simulink model "PubIfDecisionTOS_MDL"  (R2020b)
settings: configuration reference "DspaceConfig" (kept outside this file)
PostLoadFcn:
  | if any(exist('dsrtsu_mdlpostloadfcn', 'file') ~= 0), dsrtsu_mdlpostloadfcn('Execute', bdroot); end
InitFcn:
  | , if any(exist('dsmpb_private', 'file') ~= 0), dsmpb_private('dsmpb_mdlclblib', 'Init', bdroot); end,
undefined symbols (not defined in the file or in its folder): C_TOS_ACCEgoRAxletoFbumplength_m, C_TOS_ACCTargetFront_Flag, C_TOS_AEBJAPedObjDxThre_Val, C_TOS_AEBJAPedObjDyThre_Val, C_TOS_AEBJATargetSize_Val, C_TOS_AEBJAVehObjDxThre_Val, C_TOS_AEBJAVehObjDyThre_Val, C_TOS_AEBJuncPedTargetSize_Val, C_TOS_AEBLatObjDxThre_Val, C_TOS_AEBLatPedDyThre_Val, C_TOS_AEBLatTargetSize_Val, C_TOS_AEBLongTargetInEgoFront_Flag, C_TOS_axAbsGround_Parameter, C_TOS_CameraConfirmedFlag, C_TOS_CNsubjWidth, C_TOS_CurrentLaneCoreMinWidth_Val, C_TOS_CutInProb_Val_Zero, C_TOS_CutOutProb_Val_Zero, C_TOS_D2R_Val, C_TOS_DefaultValueObjectToCenterLine_dy, C_TOS_EgoCarWidth_Val, C_TOS_EgoDxRefPoint_m, C_TOS_EgoRAxletoFbumplength_m, C_TOS_HalfWidthVehicle_Con, C_TOS_HWA_CurrentLaneFlag, C_TOS_HWA_LeftLaneFlag, C_TOS_HWA_MovingDir_Vaild, C_TOS_HWA_MovState_Vaild, C_TOS_HWA_RightLaneFlag, C_TOS_LaneLineCourseErrorFront, C_TOS_LaneLineCourseErrorRear, C_TOS_MotorbikeDefaultWidth_m, C_TOS_NumberOfEffectiveTargets, C_TOS_Obj_Age_Val, C_TOS_Objdx_Constraint_Val, C_TOS_ObjectDefaultWidth_m, C_TOS_ObjInCurrentLane_Val, C_TOS_ObjInCurrentLaneValid, C_TOS_ObjInLeftLaneValid, C_TOS_ObjInRightLaneValid, C_TOS_ObjNotInCurrentLane_Val, C_TOS_ObjNotREElementType, C_TOS_ObjPredictDis_dy_ConstantVal_Zeros, C_TOS_ObjToCenterLine_ConstantVal_Zeros, C_TOS_OFMObjIDInvilad_Val, C_TOS_PIL_LatDisCons_Val_zero, C_TOS_PIL_ObjectCutInFlag_b, C_TOS_PIL_ObjectCutOutFlag_b, C_TOS_PIL_ObjLaneProb_al_Val, C_TOS_PP_ObjFusType_FC_Confirm_b, C_TOS_PP_ObjFusType_FC_FR_Confirm_b, C_TOS_PP_ObjFusType_FR_Confirm_b, C_TOS_RE_80BoolDefault_Val, C_TOS_RE_80Single181Default_Val, C_TOS_RE_80Single255Default_Val, C_TOS_RE_80Uint8Default_Val, C_TOS_RE_D2R, C_TOS_RE_D_180_Val, C_TOS_RE_InvalidObjectID_Val, C_TOS_RE_InvalidTargetChainDir_Val ... (+142)
libraries: simulink x1650, TOS_LIB x361, canfdmsglib x14
(part 60 of 69)

== system PubIfDecisionTOS_MDL/TOS_20201112/TOS_2012080320/TOS/AEB/TOS_AEBLong/AEBLong_Confirm/AEBLong/AEBLong_TrgConfirm/AEBLongTrgJudg/TOS_AEBLong_TargetMovingDir/ObjMovingDirSignalProcessing1/Oncoming_MovingDir_StrightLane/OncomingVYCondition ==
  Object_MappingVY : Inport
  Object_MappingVX : Inport  Port=2
  Abs : Abs
  Abs1 : Abs
  Relational Operator : RelationalOperator  Operator=<  OutDataTypeStr=boolean  RndMeth=Nearest
  VYThre_BaseVX : Lookup_n-D  NumberOfTableDimensions=1  BreakpointsForDimension1=[0,8.3,16.67,25,33.3,40]  Table=[0,3.5,5,7.5,9.3,9.3]  InternalRulePriority=Speed  RndMeth=Simplest  InputSameDT=on
  OncomingVYflg : Outport
  wires:
  Object_MappingVX/1 -> Abs1/1
  Relational Operator/1 -> OncomingVYflg/1
  Abs/1 -> Relational Operator/1
  VYThre_BaseVX/1 -> Relational Operator/2
  Object_MappingVY/1 -> Abs/1
  Abs1/1 -> VYThre_BaseVX/1

== system PubIfDecisionTOS_MDL/TOS_20201112/TOS_2012080320/TOS/AEB/TOS_AEBLong/AEBLong_Confirm/AEBLong/AEBLong_TrgConfirm/AEBLongTrgJudg/TOS_AEBLong_TargetMovingDir/ObjMovingDirSignalProcessing1/Oncoming_MovingDir_StrightLane/OncomingVYVXAngle ==
  Object_VXVYAngle : Inport
  135 : Constant  Value=P_TOS_ObjLatCroYawAngMaxThre_Val  OutDataTypeStr=single
      settings: AttributesFormatString=P_TOS_ObjLatCroYawAngMaxThre_Val = 135
  45 : Constant  Value=P_TOS_ObjOncomingYawAngMaxThre_Val  OutDataTypeStr=single
      settings: AttributesFormatString=P_TOS_ObjOncomingYawAngMaxThre_Val = 180
  Abs : Abs
  Logical Operator : Logic  AllPortsSameDT=off  OutDataTypeStr=boolean
  Relational Operator : RelationalOperator  Operator=>  OutDataTypeStr=boolean  RndMeth=Nearest
  Relational Operator1 : RelationalOperator  Operator=<=  OutDataTypeStr=boolean  RndMeth=Nearest
  OncomingVYVXAngleFlg : Outport
  wires:
  Logical Operator/1 -> OncomingVYVXAngleFlg/1
  Relational Operator1/1 -> Logical Operator/2
  45/1 -> Relational Operator1/2
  135/1 -> Relational Operator/2
  Abs/1 -> Relational Operator1/1, Relational Operator/1
  Relational Operator/1 -> Logical Operator/1
  Object_VXVYAngle/1 -> Abs/1

== system PubIfDecisionTOS_MDL/TOS_20201112/TOS_2012080320/TOS/AEB/TOS_AEBLong/AEBLong_Confirm/AEBLong/AEBLong_TrgConfirm/AEBLongTrgJudg/TOS_AEBLong_TargetMovingDir/ObjMovingDirSignalProcessing1/Oncoming_MovingDir_StrightLane1/CrossingVXCondition ==
  Object_MappingVX : Inport
  Object_MappingVY : Inport  Port=2
  Abs : Abs
  Abs1 : Abs
  Relational Operator : RelationalOperator  Operator=<  OutDataTypeStr=boolean  RndMeth=Nearest
  VXThre_BaseVY : Lookup_n-D  NumberOfTableDimensions=1  BreakpointsForDimension1=[0,8.3,16.67,25,33.3,40]  Table=[0,2.1,4.5,6.7,9,9]  InternalRulePriority=Speed  RndMeth=Simplest  InputSameDT=on
  CrossingVXflg : Outport
  wires:
  Object_MappingVX/1 -> Abs/1
  VXThre_BaseVY/1 -> Relational Operator/2
  Abs/1 -> Relational Operator/1
  Relational Operator/1 -> CrossingVXflg/1
  Object_MappingVY/1 -> Abs1/1
  Abs1/1 -> VXThre_BaseVY/1

== system PubIfDecisionTOS_MDL/TOS_20201112/TOS_2012080320/TOS/AEB/TOS_AEBLong/AEBLong_Confirm/AEBLong/AEBLong_TrgConfirm/AEBLongTrgJudg/TOS_AEBLong_TargetMovingDir/ObjMovingDirSignalProcessing1/Oncoming_MovingDir_StrightLane1/CrossingVYCondition ==
  note: VYThre
  Object_MappingVY : Inport
  Object_DX : Inport  Port=2
  Object_DY : Inport  Port=3
  Abs : Abs
  Abs1 : Abs
  Abs2 : Abs
  Product : Product
  Relational Operator1 : RelationalOperator  Operator=>  OutDataTypeStr=boolean  RndMeth=Nearest
  VYThre_BaseDX : Lookup_n-D  NumberOfTableDimensions=1  BreakpointsForDimension1=[0,30,60,90,120,150]  Table=[0,0.5,0.7,0.8,0.9,0.9]  InternalRulePriority=Speed  RndMeth=Simplest  InputSameDT=on
  VYThre_BaseDY : Lookup_n-D  NumberOfTableDimensions=1  BreakpointsForDimension1=[0,5,10,15,20,30,50]  Table=[1,1.1,1.12,1.15,1.2,1.2,1.2]  InternalRulePriority=Speed  RndMeth=Simplest  InputSameDT=on
  CrossingVYFlg : Outport
  wires:
  Object_MappingVY/1 -> Abs/1
  Product/1 -> Relational Operator1/2
  VYThre_BaseDX/1 -> Product/1
  Relational Operator1/1 -> CrossingVYFlg/1
  Object_DX/1 -> Abs1/1
  VYThre_BaseDY/1 -> Product/2
  Object_DY/1 -> Abs2/1
  Abs/1 -> Relational Operator1/1
  Abs1/1 -> VYThre_BaseDX/1
  Abs2/1 -> VYThre_BaseDY/1

== system PubIfDecisionTOS_MDL/TOS_20201112/TOS_2012080320/TOS/AEB/TOS_AEBLong/AEBLong_Confirm/AEBLong/AEBLong_TrgConfirm/AEBLongTrgJudg/TOS_AEBLong_TargetMovingDir/ObjMovingDirSignalProcessing1/Oncoming_MovingDir_StrightLane1/CrossingVYVXAngle ==
  Object_VYVXAngle : Inport
  135.0 : Constant  Value=P_TOS_ObjLatCroYawAngMaxThre_Val  OutDataTypeStr=single
      settings: AttributesFormatString=P_TOS_ObjLatCroYawAngMaxThre_Val = 135
  45.00 : Constant  Value=P_TOS_ObjLatCroYawAngMinThre_Val  OutDataTypeStr=single
      settings: AttributesFormatString=P_TOS_ObjLatCroYawAngMinThre_Val = 45
  Abs : Abs
  Logical Operator : Logic  AllPortsSameDT=off  OutDataTypeStr=boolean
  Relational Operator : RelationalOperator  Operator=>  OutDataTypeStr=boolean  RndMeth=Nearest
  Relational Operator1 : RelationalOperator  Operator=<=  OutDataTypeStr=boolean  RndMeth=Nearest
  CrossingVYVXAngleFlg : Outport
  wires:
  Object_VYVXAngle/1 -> Abs/1
  Relational Operator/1 -> Logical Operator/1
  Abs/1 -> Relational Operator/1, Relational Operator1/1
  45.00/1 -> Relational Operator/2
  135.0/1 -> Relational Operator1/2
  Relational Operator1/1 -> Logical Operator/2
  Logical Operator/1 -> CrossingVYVXAngleFlg/1

== system PubIfDecisionTOS_MDL/TOS_20201112/TOS_2012080320/TOS/LC_LCKie_ELK/TOS_HWA/CurrentLane/HWA_CurrentLane_Target/HWA_CLF_Target_1/HWA_CLF_Target/HWA_CLF_Target/HWA_CLF_FusionTypeConfirm/TOS_ACCFusionTypeAborDly/If Action Subsystem ==
  HWA_CLF_FusionType : Inport
  Action Port : ActionPort  ActionPortLabel=else
  HWA_CLF_FusionTypeFilt : Outport
  wires:
  HWA_CLF_FusionType/1 -> HWA_CLF_FusionTypeFilt/1

== system PubIfDecisionTOS_MDL/TOS_20201112/TOS_2012080320/TOS/LC_LCKie_ELK/TOS_HWA/CurrentLane/HWA_CurrentLane_Target/HWA_CLF_Target_1/HWA_CLF_Target/HWA_CLF_Target/HWA_CLF_FusionTypeConfirm/TOS_ACCFusionTypeAborDly/If Action Subsystem1 ==
  HWA_CLF_FusionType : Inport
  Action Port : ActionPort  ActionPortLabel=if(u1)
  Constant : Constant  Value=0.15
  Constant4 : Constant  Value=0.05
  StateDelayAbortion : TOS_LIB/StateDelayAbortion  SystemSampleTime=-1  VariantActivationTime=update diagram  Latency=0  AutoFrameSizeCalculation=off
  HWA_CLF_FusionTypeFilt : Outport
  wires:
  StateDelayAbortion/1 -> HWA_CLF_FusionTypeFilt/1
  Constant/1 -> StateDelayAbortion/2
  Constant4/1 -> StateDelayAbortion/3
  HWA_CLF_FusionType/1 -> StateDelayAbortion/1

== system PubIfDecisionTOS_MDL/TOS_20201112/TOS_2012080320/TOS/LC_LCKie_ELK/TOS_HWA/CurrentLane/HWA_CurrentLane_Target/HWA_CLF_Target_1/HWA_CLF_Target/HWA_CLF_Target/HWA_CLF_ObjTypeConfirm/TOS_ObjTypeAborDly/If Action Subsystem ==
  FusionType : Inport
  Action Port : ActionPort  ActionPortLabel=else
  FusionTypeFilt : Outport
  wires:
  FusionType/1 -> FusionTypeFilt/1

== system PubIfDecisionTOS_MDL/TOS_20201112/TOS_2012080320/TOS/LC_LCKie_ELK/TOS_HWA/CurrentLane/HWA_CurrentLane_Target/HWA_CLF_Target_1/HWA_CLF_Target/HWA_CLF_Target/HWA_CLF_ObjTypeConfirm/TOS_ObjTypeAborDly/If Action Subsystem1 ==
  FusionType : Inport
  Action Port : ActionPort  ActionPortLabel=if(u1)
  Constant : Constant  Value=0.15
  Constant4 : Constant  Value=0.05
  StateDelayAbortion : TOS_LIB/StateDelayAbortion  SystemSampleTime=-1  VariantActivationTime=update diagram  Latency=0  AutoFrameSizeCalculation=off
  FusionTypeFilt : Outport
  wires:
  StateDelayAbortion/1 -> FusionTypeFilt/1
  Constant/1 -> StateDelayAbortion/2
  Constant4/1 -> StateDelayAbortion/3
  FusionType/1 -> StateDelayAbortion/1

== system PubIfDecisionTOS_MDL/TOS_20201112/TOS_2012080320/TOS/LC_LCKie_ELK/TOS_HWA/CurrentLane/HWA_CurrentLane_Target/HWA_CLF_Target_1/HWA_CLF_Target/HWA_CLF_Target/HWA_CLF_ObstacleProbConfirm/ObstacleProbAborDly/If Action Subsystem ==
  FusionType : Inport
  Action Port : ActionPort  ActionPortLabel=else
  FusionTypeFilt : Outport
  wires:
  FusionType/1 -> FusionTypeFilt/1

== system PubIfDecisionTOS_MDL/TOS_20201112/TOS_2012080320/TOS/LC_LCKie_ELK/TOS_HWA/CurrentLane/HWA_CurrentLane_Target/HWA_CLF_Target_1/HWA_CLF_Target/HWA_CLF_Target/HWA_CLF_ObstacleProbConfirm/ObstacleProbAborDly/If Action Subsystem1 ==
  FusionType : Inport
  Action Port : ActionPort  ActionPortLabel=if(u1)
  Constant : Constant  Value=0.15
  Constant4 : Constant  Value=0.05
  StateDelayAbortion : TOS_LIB/StateDelayAbortion  SystemSampleTime=-1  VariantActivationTime=update diagram  Latency=0  AutoFrameSizeCalculation=off
  FusionTypeFilt : Outport
  wires:
  StateDelayAbortion/1 -> FusionTypeFilt/1
  Constant/1 -> StateDelayAbortion/2
  Constant4/1 -> StateDelayAbortion/3
  FusionType/1 -> StateDelayAbortion/1

== system PubIfDecisionTOS_MDL/TOS_20201112/TOS_2012080320/TOS/LC_LCKie_ELK/TOS_HWA/CurrentLane/HWA_CurrentLane_Target/HWA_CLF_Target_1/HWA_CLF_Target/HWA_CLF_Target/HWA_CLF_ObstacleProbConfirm/ObstacleProbAborDly/Subsystem ==
  TargetP0_ID_K1 : Inport
  ObjectID : Inport  Port=2
  Relational Operator : RelationalOperator  Operator===  OutDataTypeStr=boolean  RndMeth=Simplest
  SameTargetP0 : Outport
  wires:
  ObjectID/1 -> Relational Operator/2
  Relational Operator/1 -> SameTargetP0/1
  TargetP0_ID_K1/1 -> Relational Operator/1

== system PubIfDecisionTOS_MDL/TOS_20201112/TOS_2012080320/TOS/LC_LCKie_ELK/TOS_HWA/CurrentLane/HWA_CurrentLane_Target/HWA_CLF_Target_1/HWA_CLF_Target/HWA_CLF_Target/HWA_CLF_TargetMovingDirConfirm/HWA_MovingDirAborDly/If Action Subsystem ==
  TOS_MovingDir : Inport
  Action Port : ActionPort  ActionPortLabel=else
  TOS_MovingDirFilt : Outport
  wires:
  TOS_MovingDir/1 -> TOS_MovingDirFilt/1

== system PubIfDecisionTOS_MDL/TOS_20201112/TOS_2012080320/TOS/LC_LCKie_ELK/TOS_HWA/CurrentLane/HWA_CurrentLane_Target/HWA_CLF_Target_1/HWA_CLF_Target/HWA_CLF_Target/HWA_CLF_TargetMovingDirConfirm/HWA_MovingDirAborDly/If Action Subsystem1 ==
  TOS_MovingDir : Inport
  Action Port : ActionPort  ActionPortLabel=if(u1)
  Constant : Constant  Value=0.15
  Constant4 : Constant  Value=0.05
  StateDelayAbortion : TOS_LIB/StateDelayAbortion  SystemSampleTime=-1  VariantActivationTime=update diagram  Latency=0  AutoFrameSizeCalculation=off
  TOS_MovingDirFilt : Outport
  wires:
  StateDelayAbortion/1 -> TOS_MovingDirFilt/1
  Constant/1 -> StateDelayAbortion/2
  Constant4/1 -> StateDelayAbortion/3
  TOS_MovingDir/1 -> StateDelayAbortion/1

== system PubIfDecisionTOS_MDL/TOS_20201112/TOS_2012080320/TOS/LC_LCKie_ELK/TOS_HWA/CurrentLane/HWA_CurrentLane_Target/HWA_CLF_Target_1/HWA_CLF_Target/HWA_CLF_Target/HWA_CLF_TargetMovingDirConfirm/HWA_MovingDirAborDly/Subsystem ==
  ACC_TargetP0_ID_K1 : Inport
  ObjectID : Inport  Port=2
  Relational Operator : RelationalOperator  Operator===  OutDataTypeStr=boolean  RndMeth=Simplest
  ACC_SameTargetP0 : Outport
  wires:
  ObjectID/1 -> Relational Operator/2
  Relational Operator/1 -> ACC_SameTargetP0/1
  ACC_TargetP0_ID_K1/1 -> Relational Operator/1

== system PubIfDecisionTOS_MDL/TOS_20201112/TOS_2012080320/TOS/LC_LCKie_ELK/TOS_HWA/CurrentLane/HWA_CurrentLane_Target/HWA_CLF_Target_2/HWA_CLF_Target/HWA_CLF_Target/HWA_CLF_FusionTypeConfirm/TOS_ACCFusionTypeAborDly/If Action Subsystem ==
  HWA_CLF_FusionType : Inport
  Action Port : ActionPort  ActionPortLabel=else
  HWA_CLF_FusionTypeFilt : Outport
  wires:
  HWA_CLF_FusionType/1 -> HWA_CLF_FusionTypeFilt/1

== system PubIfDecisionTOS_MDL/TOS_20201112/TOS_2012080320/TOS/LC_LCKie_ELK/TOS_HWA/CurrentLane/HWA_CurrentLane_Target/HWA_CLF_Target_2/HWA_CLF_Target/HWA_CLF_Target/HWA_CLF_FusionTypeConfirm/TOS_ACCFusionTypeAborDly/If Action Subsystem1 ==
  HWA_CLF_FusionType : Inport
  Action Port : ActionPort  ActionPortLabel=if(u1)
  Constant : Constant  Value=0.15
  Constant4 : Constant  Value=0.05
  StateDelayAbortion : TOS_LIB/StateDelayAbortion  SystemSampleTime=-1  VariantActivationTime=update diagram  Latency=0  AutoFrameSizeCalculation=off
  HWA_CLF_FusionTypeFilt : Outport
  wires:
  HWA_CLF_FusionType/1 -> StateDelayAbortion/1
  Constant4/1 -> StateDelayAbortion/3
  Constant/1 -> StateDelayAbortion/2
  StateDelayAbortion/1 -> HWA_CLF_FusionTypeFilt/1

== system PubIfDecisionTOS_MDL/TOS_20201112/TOS_2012080320/TOS/LC_LCKie_ELK/TOS_HWA/CurrentLane/HWA_CurrentLane_Target/HWA_CLF_Target_2/HWA_CLF_Target/HWA_CLF_Target/HWA_CLF_ObjTypeConfirm/TOS_ObjTypeAborDly/If Action Subsystem ==
  FusionType : Inport
  Action Port : ActionPort  ActionPortLabel=else
  FusionTypeFilt : Outport
  wires:
  FusionType/1 -> FusionTypeFilt/1

== system PubIfDecisionTOS_MDL/TOS_20201112/TOS_2012080320/TOS/LC_LCKie_ELK/TOS_HWA/CurrentLane/HWA_CurrentLane_Target/HWA_CLF_Target_2/HWA_CLF_Target/HWA_CLF_Target/HWA_CLF_ObjTypeConfirm/TOS_ObjTypeAborDly/If Action Subsystem1 ==
  FusionType : Inport
  Action Port : ActionPort  ActionPortLabel=if(u1)
  Constant : Constant  Value=0.15
  Constant4 : Constant  Value=0.05
  StateDelayAbortion : TOS_LIB/StateDelayAbortion  SystemSampleTime=-1  VariantActivationTime=update diagram  Latency=0  AutoFrameSizeCalculation=off
  FusionTypeFilt : Outport
  wires:
  FusionType/1 -> StateDelayAbortion/1
  Constant4/1 -> StateDelayAbortion/3
  Constant/1 -> StateDelayAbortion/2
  StateDelayAbortion/1 -> FusionTypeFilt/1

== system PubIfDecisionTOS_MDL/TOS_20201112/TOS_2012080320/TOS/LC_LCKie_ELK/TOS_HWA/CurrentLane/HWA_CurrentLane_Target/HWA_CLF_Target_2/HWA_CLF_Target/HWA_CLF_Target/HWA_CLF_ObstacleProbConfirm/ObstacleProbAborDly/If Action Subsystem ==
  FusionType : Inport
  Action Port : ActionPort  ActionPortLabel=else
  FusionTypeFilt : Outport
  wires:
  FusionType/1 -> FusionTypeFilt/1

== system PubIfDecisionTOS_MDL/TOS_20201112/TOS_2012080320/TOS/LC_LCKie_ELK/TOS_HWA/CurrentLane/HWA_CurrentLane_Target/HWA_CLF_Target_2/HWA_CLF_Target/HWA_CLF_Target/HWA_CLF_ObstacleProbConfirm/ObstacleProbAborDly/If Action Subsystem1 ==
  FusionType : Inport
  Action Port : ActionPort  ActionPortLabel=if(u1)
  Constant : Constant  Value=0.15
  Constant4 : Constant  Value=0.05
  StateDelayAbortion : TOS_LIB/StateDelayAbortion  SystemSampleTime=-1  VariantActivationTime=update diagram  Latency=0  AutoFrameSizeCalculation=off
  FusionTypeFilt : Outport
  wires:
  FusionType/1 -> StateDelayAbortion/1
  Constant4/1 -> StateDelayAbortion/3
  Constant/1 -> StateDelayAbortion/2
  StateDelayAbortion/1 -> FusionTypeFilt/1

== system PubIfDecisionTOS_MDL/TOS_20201112/TOS_2012080320/TOS/LC_LCKie_ELK/TOS_HWA/CurrentLane/HWA_CurrentLane_Target/HWA_CLF_Target_2/HWA_CLF_Target/HWA_CLF_Target/HWA_CLF_ObstacleProbConfirm/ObstacleProbAborDly/Subsystem ==
  TargetP0_ID_K1 : Inport
  ObjectID : Inport  Port=2
  Relational Operator : RelationalOperator  Operator===  OutDataTypeStr=boolean  RndMeth=Simplest
  SameTargetP0 : Outport
  wires:
  TargetP0_ID_K1/1 -> Relational Operator/1
  Relational Operator/1 -> SameTargetP0/1
  ObjectID/1 -> Relational Operator/2

== system PubIfDecisionTOS_MDL/TOS_20201112/TOS_2012080320/TOS/LC_LCKie_ELK/TOS_HWA/CurrentLane/HWA_CurrentLane_Target/HWA_CLF_Target_2/HWA_CLF_Target/HWA_CLF_Target/HWA_CLF_TargetMovingDirConfirm/HWA_MovingDirAborDly/If Action Subsystem ==
  TOS_MovingDir : Inport
  Action Port : ActionPort  ActionPortLabel=else
  TOS_MovingDirFilt : Outport
  wires:
  TOS_MovingDir/1 -> TOS_MovingDirFilt/1

== system PubIfDecisionTOS_MDL/TOS_20201112/TOS_2012080320/TOS/LC_LCKie_ELK/TOS_HWA/CurrentLane/HWA_CurrentLane_Target/HWA_CLF_Target_2/HWA_CLF_Target/HWA_CLF_Target/HWA_CLF_TargetMovingDirConfirm/HWA_MovingDirAborDly/If Action Subsystem1 ==
  TOS_MovingDir : Inport
  Action Port : ActionPort  ActionPortLabel=if(u1)
  Constant : Constant  Value=0.15
  Constant4 : Constant  Value=0.05
  StateDelayAbortion : TOS_LIB/StateDelayAbortion  SystemSampleTime=-1  VariantActivationTime=update diagram  Latency=0  AutoFrameSizeCalculation=off
  TOS_MovingDirFilt : Outport
  wires:
  TOS_MovingDir/1 -> StateDelayAbortion/1
  Constant4/1 -> StateDelayAbortion/3
  Constant/1 -> StateDelayAbortion/2
  StateDelayAbortion/1 -> TOS_MovingDirFilt/1

== system PubIfDecisionTOS_MDL/TOS_20201112/TOS_2012080320/TOS/LC_LCKie_ELK/TOS_HWA/CurrentLane/HWA_CurrentLane_Target/HWA_CLF_Target_2/HWA_CLF_Target/HWA_CLF_Target/HWA_CLF_TargetMovingDirConfirm/HWA_MovingDirAborDly/Subsystem ==
  ACC_TargetP0_ID_K1 : Inport
  ObjectID : Inport  Port=2
  Relational Operator : RelationalOperator  Operator===  OutDataTypeStr=boolean  RndMeth=Simplest
  ACC_SameTargetP0 : Outport
  wires:
  ACC_TargetP0_ID_K1/1 -> Relational Operator/1
  Relational Operator/1 -> ACC_SameTargetP0/1
  ObjectID/1 -> Relational Operator/2

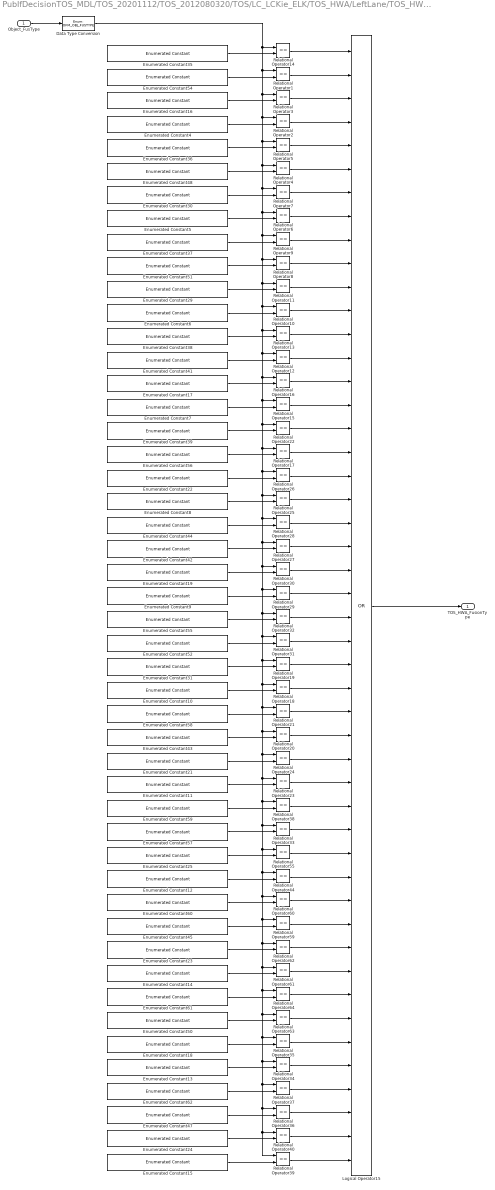
== system PubIfDecisionTOS_MDL/TOS_20201112/TOS_2012080320/TOS/LC_LCKie_ELK/TOS_HWA/LeftLane/TOS_HWA_LeftLane/TOS_HWA_LeftLane/TOS_HWA/HWA_LeftLane/HWA_LeftLane_Rear/HWA_LeftRear_FusionType/FusionType ==
  Object_FusType : Inport
  Data Type Conversion : DataTypeConversion  OutDataTypeStr=Enum: OFM_OBJ_FUSTYPE
  Enumerated Constant10 : simulink/Sources/Enumerated Constant  OutDataTypeStr=Enum: OFM_OBJ_FUSTYPE  Value=OFM_OBJ_FUSTYPE.FC_FR_CR_BR  SampleTime=inf
      settings: AttributesFormatString=OFM_OBJ_FUSTYPE.FC_FR_CR_BR=43
  Enumerated Constant11 : simulink/Sources/Enumerated Constant  OutDataTypeStr=Enum: OFM_OBJ_FUSTYPE  Value=OFM_OBJ_FUSTYPE.FC_FR_CL_CR_BR  SampleTime=inf
      settings: AttributesFormatString=OFM_OBJ_FUSTYPE.FC_FR_CL_CR_BR=47
  Enumerated Constant12 : simulink/Sources/Enumerated Constant  OutDataTypeStr=Enum: OFM_OBJ_FUSTYPE  Value=OFM_OBJ_FUSTYPE.FC_FR_BL_BR  SampleTime=inf
      settings: AttributesFormatString=OFM_OBJ_FUSTYPE.FC_FR_BL_BR=51
  Enumerated Constant13 : simulink/Sources/Enumerated Constant  OutDataTypeStr=Enum: OFM_OBJ_FUSTYPE  Value=OFM_OBJ_FUSTYPE.FC_FR_CR_BL_BR  SampleTime=inf
      settings: AttributesFormatString=OFM_OBJ_FUSTYPE.FC_FR_CR_BL_BR=59
  Enumerated Constant14 : simulink/Sources/Enumerated Constant  OutDataTypeStr=Enum: OFM_OBJ_FUSTYPE  Value=OFM_OBJ_FUSTYPE.FC_FR_CL_BL_BR  SampleTime=inf
      settings: AttributesFormatString=OFM_OBJ_FUSTYPE.FC_FR_CL_BL_BR=55
  Enumerated Constant15 : simulink/Sources/Enumerated Constant  OutDataTypeStr=Enum: OFM_OBJ_FUSTYPE  Value=OFM_OBJ_FUSTYPE.FC_FR_CL_CR_BL_BR  SampleTime=inf
      settings: AttributesFormatString=OFM_OBJ_FUSTYPE.FC_FR_CL_CR_BL_BR=63
  Enumerated Constant16 : simulink/Sources/Enumerated Constant  OutDataTypeStr=Enum: OFM_OBJ_FUSTYPE  Value=OFM_OBJ_FUSTYPE.FR_BL  SampleTime=inf
      settings: AttributesFormatString=OFM_OBJ_FUSTYPE.FR_BL = 18
  Enumerated Constant17 : simulink/Sources/Enumerated Constant  OutDataTypeStr=Enum: OFM_OBJ_FUSTYPE  Value=OFM_OBJ_FUSTYPE.FR_CL_CR_BL  SampleTime=inf
      settings: AttributesFormatString=OFM_OBJ_FUSTYPE.FR_CL_CR_BL = 30
  Enumerated Constant18 : simulink/Sources/Enumerated Constant  OutDataTypeStr=Enum: OFM_OBJ_FUSTYPE  Value=OFM_OBJ_FUSTYPE.FR_CR_BL_BR  SampleTime=inf
      settings: AttributesFormatString=OFM_OBJ_FUSTYPE.FR_CR_BL_BR = 58
  Enumerated Constant19 : simulink/Sources/Enumerated Constant  OutDataTypeStr=Enum: OFM_OBJ_FUSTYPE  Value=OFM_OBJ_FUSTYPE.FR_CL_BR  SampleTime=inf
      settings: AttributesFormatString=OFM_OBJ_FUSTYPE.FR_CL_BR = 38
  Enumerated Constant21 : simulink/Sources/Enumerated Constant  OutDataTypeStr=Enum: OFM_OBJ_FUSTYPE  Value=OFM_OBJ_FUSTYPE.FR_CL_CR_BR  SampleTime=inf
      settings: AttributesFormatString=OFM_OBJ_FUSTYPE.FR_CL_CR_BR = 46
  Enumerated Constant22 : simulink/Sources/Enumerated Constant  OutDataTypeStr=Enum: OFM_OBJ_FUSTYPE  Value=OFM_OBJ_FUSTYPE.FR_BR  SampleTime=inf
      settings: AttributesFormatString=OFM_OBJ_FUSTYPE.FR_BR = 34
  Enumerated Constant23 : simulink/Sources/Enumerated Constant  OutDataTypeStr=Enum: OFM_OBJ_FUSTYPE  Value=OFM_OBJ_FUSTYPE.FR_CL_BL_BR  SampleTime=inf
      settings: AttributesFormatString=OFM_OBJ_FUSTYPE.FR_CL_BL_BR = 54
  Enumerated Constant24 : simulink/Sources/Enumerated Constant  OutDataTypeStr=Enum: OFM_OBJ_FUSTYPE  Value=OFM_OBJ_FUSTYPE.FR_CL_CR_BL_BR  SampleTime=inf
      settings: AttributesFormatString=OFM_OBJ_FUSTYPE.FR_CL_CR_BL_BR = 62
  Enumerated Constant25 : simulink/Sources/Enumerated Constant  OutDataTypeStr=Enum: OFM_OBJ_FUSTYPE  Value=OFM_OBJ_FUSTYPE.FR_BL_BR  SampleTime=inf
      settings: AttributesFormatString=OFM_OBJ_FUSTYPE.FR_BL_BR = 50
  Enumerated Constant29 : simulink/Sources/Enumerated Constant  OutDataTypeStr=Enum: OFM_OBJ_FUSTYPE  Value=OFM_OBJ_FUSTYPE.FR_CR_BL  SampleTime=inf
      settings: AttributesFormatString=OFM_OBJ_FUSTYPE.FR_CR_BL = 26
  Enumerated Constant30 : simulink/Sources/Enumerated Constant  OutDataTypeStr=Enum: OFM_OBJ_FUSTYPE  Value=OFM_OBJ_FUSTYPE.FR_CL_BL  SampleTime=inf
      settings: AttributesFormatString=OFM_OBJ_FUSTYPE.FR_CL_BL = 22
  Enumerated Constant31 : simulink/Sources/Enumerated Constant  OutDataTypeStr=Enum: OFM_OBJ_FUSTYPE  Value=OFM_OBJ_FUSTYPE.FR_CR_BR  SampleTime=inf
      settings: AttributesFormatString=OFM_OBJ_FUSTYPE.FR_CR_BR = 42
  Enumerated Constant35 : simulink/Sources/Enumerated Constant  OutDataTypeStr=Enum: OFM_OBJ_FUSTYPE  Value=OFM_OBJ_FUSTYPE.BL  SampleTime=inf
      settings: AttributesFormatString=OFM_OBJ_FUSTYPE.BL = 16
  Enumerated Constant36 : simulink/Sources/Enumerated Constant  OutDataTypeStr=Enum: OFM_OBJ_FUSTYPE  Value=OFM_OBJ_FUSTYPE.CL_BL  SampleTime=inf
      settings: AttributesFormatString=OFM_OBJ_FUSTYPE.CL_BL=20
  Enumerated Constant37 : simulink/Sources/Enumerated Constant  OutDataTypeStr=Enum: OFM_OBJ_FUSTYPE  Value=OFM_OBJ_FUSTYPE.CR_BL  SampleTime=inf
      settings: AttributesFormatString=OFM_OBJ_FUSTYPE.CR_BL = 24
  Enumerated Constant38 : simulink/Sources/Enumerated Constant  OutDataTypeStr=Enum: OFM_OBJ_FUSTYPE  Value=OFM_OBJ_FUSTYPE.CL_CR_BL  SampleTime=inf
      settings: AttributesFormatString=OFM_OBJ_FUSTYPE.CL_CR_BL=28
  Enumerated Constant39 : simulink/Sources/Enumerated Constant  OutDataTypeStr=Enum: OFM_OBJ_FUSTYPE  Value=OFM_OBJ_FUSTYPE.BR  SampleTime=inf
      settings: AttributesFormatString=OFM_OBJ_FUSTYPE.BR = 32
  Enumerated Constant4 : simulink/Sources/Enumerated Constant  OutDataTypeStr=Enum: OFM_OBJ_FUSTYPE  Value=OFM_OBJ_FUSTYPE.FC_FR_BL  SampleTime=inf
      settings: AttributesFormatString=OFM_OBJ_FUSTYPE.FC_FR_BL=19
  Enumerated Constant41 : simulink/Sources/Enumerated Constant  OutDataTypeStr=Enum: OFM_OBJ_FUSTYPE  Value=OFM_OBJ_FUSTYPE.FC_CL_CR_BL  SampleTime=inf
      settings: AttributesFormatString=OFM_OBJ_FUSTYPE.FC_CL_CR_BL = 29
  Enumerated Constant42 : simulink/Sources/Enumerated Constant  OutDataTypeStr=Enum: OFM_OBJ_FUSTYPE  Value=OFM_OBJ_FUSTYPE.FC_CL_BR  SampleTime=inf
      settings: AttributesFormatString=OFM_OBJ_FUSTYPE.FC_CL_BR = 37
  Enumerated Constant43 : simulink/Sources/Enumerated Constant  OutDataTypeStr=Enum: OFM_OBJ_FUSTYPE  Value=OFM_OBJ_FUSTYPE.FC_CL_CR_BR  SampleTime=inf
      settings: AttributesFormatString=OFM_OBJ_FUSTYPE.FC_CL_CR_BR = 45
  Enumerated Constant44 : simulink/Sources/Enumerated Constant  OutDataTypeStr=Enum: OFM_OBJ_FUSTYPE  Value=OFM_OBJ_FUSTYPE.CL_BR  SampleTime=inf
      settings: AttributesFormatString=OFM_OBJ_FUSTYPE.CL_BR = 36
  Enumerated Constant45 : simulink/Sources/Enumerated Constant  OutDataTypeStr=Enum: OFM_OBJ_FUSTYPE  Value=OFM_OBJ_FUSTYPE.FC_CL_BL_BR  SampleTime=inf
      settings: AttributesFormatString=OFM_OBJ_FUSTYPE.FC_CL_BL_BR = 53
  Enumerated Constant47 : simulink/Sources/Enumerated Constant  OutDataTypeStr=Enum: OFM_OBJ_FUSTYPE  Value=OFM_OBJ_FUSTYPE.FC_CL_CR_BL_BR  SampleTime=inf
      settings: AttributesFormatString=OFM_OBJ_FUSTYPE.FC_CL_CR_BL_BR = 61
  Enumerated Constant48 : simulink/Sources/Enumerated Constant  OutDataTypeStr=Enum: OFM_OBJ_FUSTYPE  Value=OFM_OBJ_FUSTYPE.FC_CL_BL  SampleTime=inf
      settings: AttributesFormatString=OFM_OBJ_FUSTYPE.FC_CL_BL = 21
  Enumerated Constant5 : simulink/Sources/Enumerated Constant  OutDataTypeStr=Enum: OFM_OBJ_FUSTYPE  Value=OFM_OBJ_FUSTYPE.FC_FR_CL_BL  SampleTime=inf
      settings: AttributesFormatString=OFM_OBJ_FUSTYPE.FC_FR_CL_BL=23
  Enumerated Constant50 : simulink/Sources/Enumerated Constant  OutDataTypeStr=Enum: OFM_OBJ_FUSTYPE  Value=OFM_OBJ_FUSTYPE.FC_CR_BL_BR  SampleTime=inf
      settings: AttributesFormatString=OFM_OBJ_FUSTYPE.FC_CR_BL_BR = 57
  Enumerated Constant51 : simulink/Sources/Enumerated Constant  OutDataTypeStr=Enum: OFM_OBJ_FUSTYPE  Value=OFM_OBJ_FUSTYPE.FC_CR_BL  SampleTime=inf
      settings: AttributesFormatString=OFM_OBJ_FUSTYPE.FC_CR_BL = 25
  Enumerated Constant52 : simulink/Sources/Enumerated Constant  OutDataTypeStr=Enum: OFM_OBJ_FUSTYPE  Value=OFM_OBJ_FUSTYPE.FC_CR_BR  SampleTime=inf
      settings: AttributesFormatString=OFM_OBJ_FUSTYPE.FC_CR_BR = 41
  Enumerated Constant54 : simulink/Sources/Enumerated Constant  OutDataTypeStr=Enum: OFM_OBJ_FUSTYPE  Value=OFM_OBJ_FUSTYPE.FC_BL  SampleTime=inf
      settings: AttributesFormatString=OFM_OBJ_FUSTYPE.FC_BL = 17
  Enumerated Constant55 : simulink/Sources/Enumerated Constant  OutDataTypeStr=Enum: OFM_OBJ_FUSTYPE  Value=OFM_OBJ_FUSTYPE.CR_BR  SampleTime=inf
      settings: AttributesFormatString=OFM_OBJ_FUSTYPE.CR_BR = 40
  Enumerated Constant56 : simulink/Sources/Enumerated Constant  OutDataTypeStr=Enum: OFM_OBJ_FUSTYPE  Value=OFM_OBJ_FUSTYPE.FC_BR  SampleTime=inf
      settings: AttributesFormatString=OFM_OBJ_FUSTYPE.FC_BR = 33
  Enumerated Constant57 : simulink/Sources/Enumerated Constant  OutDataTypeStr=Enum: OFM_OBJ_FUSTYPE  Value=OFM_OBJ_FUSTYPE.FC_BL_BR  SampleTime=inf
      settings: AttributesFormatString=OFM_OBJ_FUSTYPE.FC_BL_BR = 49
  Enumerated Constant58 : simulink/Sources/Enumerated Constant  OutDataTypeStr=Enum: OFM_OBJ_FUSTYPE  Value=OFM_OBJ_FUSTYPE.CL_CR_BR  SampleTime=inf
      settings: AttributesFormatString=OFM_OBJ_FUSTYPE.CL_CR_BR = 44
  Enumerated Constant59 : simulink/Sources/Enumerated Constant  OutDataTypeStr=Enum: OFM_OBJ_FUSTYPE  Value=OFM_OBJ_FUSTYPE.BL_BR  SampleTime=inf
      settings: AttributesFormatString=OFM_OBJ_FUSTYPE.BL_BR = 48
  Enumerated Constant6 : simulink/Sources/Enumerated Constant  OutDataTypeStr=Enum: OFM_OBJ_FUSTYPE  Value=OFM_OBJ_FUSTYPE.FC_FR_CR_BL  SampleTime=inf
      settings: AttributesFormatString=OFM_OBJ_FUSTYPE.FC_FR_CR_BL=27
  Enumerated Constant60 : simulink/Sources/Enumerated Constant  OutDataTypeStr=Enum: OFM_OBJ_FUSTYPE  Value=OFM_OBJ_FUSTYPE.CL_BL_BR  SampleTime=inf
      settings: AttributesFormatString=OFM_OBJ_FUSTYPE.CL_BL_BR = 52
  Enumerated Constant61 : simulink/Sources/Enumerated Constant  OutDataTypeStr=Enum: OFM_OBJ_FUSTYPE  Value=OFM_OBJ_FUSTYPE.CR_BL_BR  SampleTime=inf
      settings: AttributesFormatString=OFM_OBJ_FUSTYPE.CR_BL_BR = 56
  Enumerated Constant62 : simulink/Sources/Enumerated Constant  OutDataTypeStr=Enum: OFM_OBJ_FUSTYPE  Value=OFM_OBJ_FUSTYPE.CL_CR_BL_BR  SampleTime=inf
      settings: AttributesFormatString=OFM_OBJ_FUSTYPE.CL_CR_BL_BR = 60
  Enumerated Constant7 : simulink/Sources/Enumerated Constant  OutDataTypeStr=Enum: OFM_OBJ_FUSTYPE  Value=OFM_OBJ_FUSTYPE.FC_FR_CL_CR_BL  SampleTime=inf
      settings: AttributesFormatString=OFM_OBJ_FUSTYPE.FC_FR_CL_CR_BL=31
  Enumerated Constant8 : simulink/Sources/Enumerated Constant  OutDataTypeStr=Enum: OFM_OBJ_FUSTYPE  Value=OFM_OBJ_FUSTYPE.FC_FR_BR  SampleTime=inf
      settings: AttributesFormatString=OFM_OBJ_FUSTYPE.FC_FR_BR=35
  Enumerated Constant9 : simulink/Sources/Enumerated Constant  OutDataTypeStr=Enum: OFM_OBJ_FUSTYPE  Value=OFM_OBJ_FUSTYPE.FC_FR_CL_BR  SampleTime=inf
      settings: AttributesFormatString=OFM_OBJ_FUSTYPE.FC_FR_CL_BR=39
  Logical Operator15 : Logic  Operator=OR  Inputs=48  AllPortsSameDT=off  OutDataTypeStr=boolean
  Relational Operator{1..40,44,55,59..64} (48 alike) : RelationalOperator  Operator===  OutDataTypeStr=boolean  RndMeth=Nearest
  TOS_HWA_FusionType : Outport
  wires:
  Relational Operator12/1 -> Logical Operator15/14
  Data Type Conversion/1 -> Relational Operator14/1, Relational Operator35/1, Relational Operator39/1, Relational Operator40/1, Relational Operator36/1, Relational Operator37/1, Relational Operator34/1, Relational Operator63/1, Relational Operator64/1, Relational Operator61/1, Relational Operator62/1, Relational Operator59/1, Relational Operator60/1, Relational Operator44/1, Relational Operator55/1, Relational Operator33/1, Relational Operator38/1, Relational Operator23/1, Relational Operator24/1, Relational Operator20/1, Relational Operator21/1, Relational Operator18/1, Relational Operator19/1, Relational Operator31/1, Relational Operator32/1, Relational Operator29/1, Relational Operator30/1, Relational Operator27/1, Relational Operator28/1, Relational Operator25/1, Relational Operator26/1, Relational Operator17/1, Relational Operator22/1, Relational Operator15/1, Relational Operator16/1, Relational Operator12/1, Relational Operator13/1, Relational Operator10/1, Relational Operator11/1, Relational Operator8/1, Relational Operator9/1, Relational Operator6/1, Relational Operator7/1, Relational Operator4/1, Relational Operator5/1, Relational Operator2/1, Relational Operator3/1, Relational Operator1/1
  Enumerated Constant39/1 -> Relational Operator22/2
  Relational Operator14/1 -> Logical Operator15/1
  Enumerated Constant36/1 -> Relational Operator5/2
  Relational Operator55/1 -> Logical Operator15/35
  Relational Operator31/1 -> Logical Operator15/26
  Enumerated Constant62/1 -> Relational Operator37/2
  Enumerated Constant42/1 -> Relational Operator27/2
  Relational Operator62/1 -> Logical Operator15/39
  Enumerated Constant17/1 -> Relational Operator16/2
  Relational Operator30/1 -> Logical Operator15/23
  Enumerated Constant10/1 -> Relational Operator18/2
  Enumerated Constant52/1 -> Relational Operator31/2
  Enumerated Constant56/1 -> Relational Operator17/2
  Enumerated Constant29/1 -> Relational Operator11/2
  Enumerated Constant51/1 -> Relational Operator8/2
  Enumerated Constant24/1 -> Relational Operator40/2
  Relational Operator39/1 -> Logical Operator15/48
  Relational Operator32/1 -> Logical Operator15/25
  Relational Operator5/1 -> Logical Operator15/5
  Object_FusType/1 -> Data Type Conversion/1
  Relational Operator37/1 -> Logical Operator15/45
  Enumerated Constant38/1 -> Relational Operator13/2
  Enumerated Constant13/1 -> Relational Operator34/2
  Enumerated Constant47/1 -> Relational Operator36/2
  Enumerated Constant8/1 -> Relational Operator25/2
  Relational Operator4/1 -> Logical Operator15/6
  Relational Operator2/1 -> Logical Operator15/4
  Relational Operator40/1 -> Logical Operator15/47
  Enumerated Constant61/1 -> Relational Operator64/2
  Enumerated Constant60/1 -> Relational Operator60/2
  Relational Operator21/1 -> Logical Operator15/29
  Relational Operator24/1 -> Logical Operator15/31
  Enumerated Constant25/1 -> Relational Operator55/2
  Relational Operator10/1 -> Logical Operator15/12
  Enumerated Constant5/1 -> Relational Operator6/2
  Enumerated Constant18/1 -> Relational Operator35/2
  Relational Operator19/1 -> Logical Operator15/27
  Relational Operator61/1 -> Logical Operator15/40
  Enumerated Constant43/1 -> Relational Operator20/2
  Enumerated Constant55/1 -> Relational Operator32/2
  Enumerated Constant31/1 -> Relational Operator19/2
  Relational Operator20/1 -> Logical Operator15/30
  Relational Operator36/1 -> Logical Operator15/46
  Enumerated Constant14/1 -> Relational Operator61/2
  Enumerated Constant11/1 -> Relational Operator23/2
  Enumerated Constant12/1 -> Relational Operator44/2
  Relational Operator18/1 -> Logical Operator15/28
  Enumerated Constant45/1 -> Relational Operator59/2
  Relational Operator60/1 -> Logical Operator15/37
  Relational Operator26/1 -> Logical Operator15/19
  Relational Operator11/1 -> Logical Operator15/11
  Enumerated Constant9/1 -> Relational Operator29/2
  Relational Operator6/1 -> Logical Operator15/8
  Enumerated Constant21/1 -> Relational Operator24/2
  Enumerated Constant59/1 -> Relational Operator38/2
  Enumerated Constant37/1 -> Relational Operator9/2
  Enumerated Constant35/1 -> Relational Operator14/2
  Relational Operator22/1 -> Logical Operator15/17
  Enumerated Constant22/1 -> Relational Operator26/2
  Relational Operator59/1 -> Logical Operator15/38
  Relational Operator15/1 -> Logical Operator15/16
  Relational Operator34/1 -> Logical Operator15/44
  Relational Operator44/1 -> Logical Operator15/36
  Enumerated Constant6/1 -> Relational Operator10/2
  Relational Operator63/1 -> Logical Operator15/42
  Relational Operator35/1 -> Logical Operator15/43
  Relational Operator64/1 -> Logical Operator15/41
  Enumerated Constant7/1 -> Relational Operator15/2
  Enumerated Constant41/1 -> Relational Operator12/2
  Relational Operator1/1 -> Logical Operator15/2
  Relational Operator25/1 -> Logical Operator15/20
  Relational Operator17/1 -> Logical Operator15/18
  Enumerated Constant30/1 -> Relational Operator7/2
  Enumerated Constant19/1 -> Relational Operator30/2
  Relational Operator33/1 -> Logical Operator15/34
  Enumerated Constant57/1 -> Relational Operator33/2
  Relational Operator9/1 -> Logical Operator15/9
  Enumerated Constant4/1 -> Relational Operator2/2
  Enumerated Constant16/1 -> Relational Operator3/2
  Relational Operator38/1 -> Logical Operator15/33
  Relational Operator3/1 -> Logical Operator15/3
  Relational Operator13/1 -> Logical Operator15/13
  Relational Operator23/1 -> Logical Operator15/32
  Logical Operator15/1 -> TOS_HWA_FusionType/1
  Relational Operator28/1 -> Logical Operator15/21
  Enumerated Constant23/1 -> Relational Operator62/2
  Enumerated Constant48/1 -> Relational Operator4/2
  Enumerated Constant44/1 -> Relational Operator28/2
  Relational Operator16/1 -> Logical Operator15/15
  Enumerated Constant58/1 -> Relational Operator21/2
  Enumerated Constant54/1 -> Relational Operator1/2
  Relational Operator7/1 -> Logical Operator15/7
  Relational Operator27/1 -> Logical Operator15/22
  Relational Operator8/1 -> Logical Operator15/10
  Enumerated Constant15/1 -> Relational Operator39/2
  Enumerated Constant50/1 -> Relational Operator63/2
  Relational Operator29/1 -> Logical Operator15/24
